simulink model "building_EXAMPLE_v2_r2018b"  (R2018b)
settings: Solver=ode23tb  StartTime=-building.preruntime+8760*3600  StopTime=building.runtime+8760*3600  MaxStep=600  EnableMultiTasking=on
StartFcn:
  | tic
StopFcn:
  | toc
values from neighbouring files (symbols this model uses):
  building = building.add_simulation(1, 'Innsbruck - ERV, 120m3/h, 230 g/h', saveAIB, saveBDB, saveBOUNDARY, saveHVAC, 1)    [work_EXAMPLE_v1.m]
undefined symbols (not defined in the file or in its folder): cp, Dreifach, get_building, p, Qdot_C, Qdot_C_energy, Qdot_H, Qdot_H_energy, Qdot_I_electricity, Qdot_I_electricity_energy, Qdot_I_light, Qdot_I_light_energy, Qdot_I_person, Qdot_I_person_energy, Qdot_S, Qdot_S_energy, Qdot_T_ground, Qdot_T_ground_energy, Qdot_T_neighbour, Qdot_T_neighbour_energy, Qdot_T_opaque, Qdot_T_opaque_energy, Qdot_T_window, Qdot_T_window_energy, Qdot_V_infiltration, Qdot_V_infiltration_energy, Qdot_V_mech, Qdot_V_mech_energy, Qdot_V_window, Qdot_V_window_energy, rho, Tc, Tr, Ts, Wärmeschutzglas, x_CO2, x_H2O, x_VOC
libraries: carnotUIBK x1879, carnot x1
(part 1 of 28)
settings Model: SimulationMode=accelerator  Creator=c8461199  LastModifiedBy=eeb
settings SolverCC: ZeroCrossAlgorithm=Adaptive
settings DataIOCC: SaveOutput=off  SignalLogging=off  DSMLogging=off  VisualizeSimOutput=off  SaveTime=off
settings OptimizationCC: UseDivisionForNetSlopeComputation=on  UseFloatMulNetSlope=on  LifeSpan=inf
settings DebuggingCC: MaxConsecutiveZCsMsg=warning  IgnoredZcDiagnostic=none  AllowSymbolicDim=off  SFUnexpectedBacktrackingDiag=warning  SFNoUnconditionalDefaultTransitionDiag=warning  SFExecutionAtInitializationDiag=none
settings ModelReferenceCC: PropagateSignalLabelsOutOfModel=off
settings SFSimCC: SimUserSources=carlib.c  SimUseLocalCustomCode=off
settings RTWCC: RTWUseLocalCustomCode=off  BuildConfiguration=Faster Runs
settings CodeAppCC: StateflowObjectComments=on
settings GRTTargetCC: TargetLangStandard=C89/C90 (ANSI)
settings ConfigComp: CovMetricSettings=dw  CovHtmlReporting=on  CovSaveCumulativeToWorkspaceVar=on  CovSaveSingleToWorkspaceVar=on  CovExternalEMLEnable=off

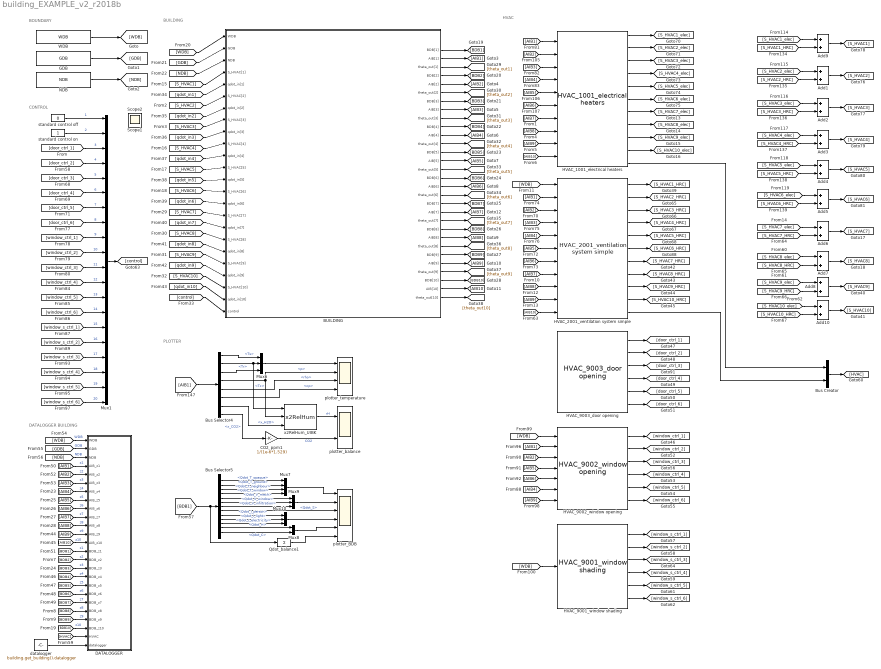
== system building_EXAMPLE_v2_r2018b ==
  note: PLOTTER
  note: DATALOGGER BUILDING
  note: BUILDING
  note: BOUNDARY
  note: HVAC
  note: CONTROL
  Add{1..10} (10 alike) : Sum  Inputs=2
  BUILDING : Subsystem  mask{building=get_building(building)}
      mask prompts: building "BUILDING object"
      mask init:
      | b = building;
      mask Display:
      | plot(-20,-30,120,100,[10,10,90,90,10],[0,50,50,0,0],...
      |     [100,60,40,0],[40,80,80,40],[20,34,34,20,20],[40,40,20,20,40],...
      |     [60,60,40,40],[0,40,40,0],[65,80,80,65,65],[40,40,20,20,40],...
      |     [47,54,54,47,47],[35,35,4,4,35],[45,41],[20,20])
  Bus Creator : BusCreator  Inputs=2
  Bus Selector4 : BusSelector  OutputSignals=Ts,Tc,Tr,p,rho,cp,x_H2O,x_CO2
  Bus Selector5 : BusSelector  OutputSignals=Qdot_T_opaque,Qdot_T_ground,Qdot_T_neighbour,Qdot_T_window,Qdot_V_mech,Qdot_V_window,Qdot_V_infiltration,Qdot_S,Qdot_I_person,Qdot_I_light,Qdot_I_electricity,Qdot_H,Qdot_C
  CO2_ppm1 : Gain  Gain=1/(1e-6*1.529)
  DATALOGGER : Subsystem
  GDB : carnotUIBK/boundary/GDB  building=get_building(building)
  HVAC_1001_electrical heaters : carnotUIBK/HVAC/HVAC_1001_electrical heaters  building=get_building(building)  system=1001
  HVAC_2001_ventilation system simple : carnotUIBK/HVAC/HVAC_2001_ventilation system simple  building=get_building(building)  system=2001
  HVAC_9001_window shading : carnotUIBK/HVAC/HVAC_9001_window shading  building=get_building(building)  system=9001
  HVAC_9002_window opening : carnotUIBK/HVAC/HVAC_9002_window opening  building=get_building(building)  system=9002
  HVAC_9003_door opening : carnotUIBK/HVAC/HVAC_9003_door opening  building=get_building(building)  system=9003
  Mux1 : Mux  Inputs=[1 1 1 1 1 1 1 1 1 1 1 1 1 1 1 1 1 1 1 1]
  Mux10 : Mux  Inputs=3
  Mux6 : Mux  Inputs=3
  Mux7 : Mux
  Mux8 : Mux  Inputs=2
  Mux9 : Mux  Inputs=3
  NDB : carnotUIBK/boundary/NDB  building=get_building(building)
  Qdot_balance1 : Sum  Inputs=1
  WDB : carnotUIBK/boundary/WDB  building=get_building(building)
  datalogger : Constant  Value=building.get_building().datalogger
  plotter_BDB : Scope  NumInputPorts=6
  plotter_balance : Scope  NumInputPorts=2
  plotter_temperature : Scope  NumInputPorts=4
  standard control off : Constant  Value=0
  standard control on : Constant
  x2RelHum_UIBK : carnot/Basic/Material_Properties/x2RelHum
  Scope1 : Scope
  Scope2 : Scope
  wires:
  WDB/1 -> [WDB]
  GDB/1 -> [GDB]
  NDB/1 -> [NDB]
  [WDB] -> BUILDING/1(WDB)
  [GDB] -> BUILDING/2(GDB)
  [NDB] -> BUILDING/3(NDB)
  BUILDING/2(AIB[1]) -> [AIB1]
  BUILDING/5(AIB[2]) -> [AIB2]
  BUILDING/8(AIB[3]) -> [AIB3]
  BUILDING/11(AIB[4]) -> [AIB4]
  BUILDING/14(AIB[5]) -> [AIB5]
  BUILDING/17(AIB[6]) -> [AIB6]
  BUILDING/29(AIB[10]) -> [AIB10]
  BUILDING/26(AIB[9]) -> [AIB9]
  BUILDING/23(AIB[8]) -> [AIB8]
  BUILDING/20(AIB[7]) -> [AIB7]
  [S_HVAC5] -> BUILDING/12(S_HVAC[5])
  [S_HVAC4] -> BUILDING/10(S_HVAC[4])
  [S_HVAC1] -> BUILDING/4(S_HVAC[1])
  [S_HVAC2] -> BUILDING/6(S_HVAC[2])
  [S_HVAC3] -> BUILDING/8(S_HVAC[3])
  [S_HVAC6] -> BUILDING/14(S_HVAC[6])
  [S_HVAC10] -> BUILDING/22(S_HVAC[10])
  [S_HVAC9] -> BUILDING/20(S_HVAC[9])
  [S_HVAC8] -> BUILDING/18(S_HVAC[8])
  [S_HVAC7] -> BUILDING/16(S_HVAC[7])
  [control] -> BUILDING/24(control)
  BUILDING/1(BDB[1]) -> [BDB1]
  BUILDING/28(BDB[10]) -> [BDB10]
  BUILDING/4(BDB[2]) -> [BDB2]
  BUILDING/7(BDB[3]) -> [BDB3]
  BUILDING/10(BDB[4]) -> [BDB4]
  BUILDING/13(BDB[5]) -> [BDB5]
  BUILDING/16(BDB[6]) -> [BDB6]
  BUILDING/19(BDB[7]) -> [BDB7]
  BUILDING/22(BDB[8]) -> [BDB8]
  BUILDING/25(BDB[9]) -> [BDB9]
  [qdot_in1] -> BUILDING/5(qdot_in[1])
  [qdot_in9] -> BUILDING/21(qdot_in[9])
  [qdot_in10] -> BUILDING/23(qdot_in[10])
  [qdot_in8] -> BUILDING/19(qdot_in[8])
  [qdot_in7] -> BUILDING/17(qdot_in[7])
  [qdot_in6] -> BUILDING/15(qdot_in[6])
  [qdot_in4] -> BUILDING/11(qdot_in[4])
  [qdot_in5] -> BUILDING/13(qdot_in[5])
  [qdot_in3] -> BUILDING/9(qdot_in[3])
  [qdot_in2] -> BUILDING/7(qdot_in[2])
  BUILDING/3(theta_out[1]) -> [theta_out1]
  BUILDING/30(theta_out[10]) -> [theta_out10]
  BUILDING/27(theta_out[9]) -> [theta_out9]
  BUILDING/24(theta_out[8]) -> [theta_out8]
  BUILDING/21(theta_out[7]) -> [theta_out7]
  BUILDING/18(theta_out[6]) -> [theta_out6]
  BUILDING/15(theta_out[5]) -> [theta_out5]
  BUILDING/12(theta_out[4]) -> [theta_out4]
  BUILDING/9(theta_out[3]) -> [theta_out3]
  BUILDING/6(theta_out[2]) -> [theta_out2]
  datalogger/1 -> DATALOGGER/25(datalogger)
  [AIB1] -> DATALOGGER/4(AIB_z1)  "z1"
  [WDB] -> DATALOGGER/1(WDB)  "WDB"
  [GDB] -> DATALOGGER/2(GDB)  "GDB"
  [NDB] -> DATALOGGER/3(NDB)  "NDB"
  [AIB2] -> DATALOGGER/5(AIB_z2)  "z2"
  [AIB3] -> DATALOGGER/6(AIB_z3)  "z3"
  [AIB4] -> DATALOGGER/7(AIB_z4)  "z4"
  [AIB5] -> DATALOGGER/8(AIB_z5)  "z5"
  [AIB6] -> DATALOGGER/9(AIB_z6)  "z6"
  [AIB7] -> DATALOGGER/10(AIB_z7)  "z7"
  [AIB8] -> DATALOGGER/11(AIB_z8)  "z8"
  [AIB9] -> DATALOGGER/12(AIB_z9)  "z9"
  [AIB10] -> DATALOGGER/13(AIB_z10)  "z10"
  [BDB1] -> DATALOGGER/14(BDB_z1)  "z1"
  [BDB2] -> DATALOGGER/15(BDB_z2)  "z2"
  [BDB3] -> DATALOGGER/16(BDB_z3)  "z3"
  [BDB4] -> DATALOGGER/17(BDB_z4)  "z4"
  [BDB5] -> DATALOGGER/18(BDB_z5)  "z5"
  [BDB6] -> DATALOGGER/19(BDB_z6)  "z6"
  [BDB7] -> DATALOGGER/20(BDB_z7)  "z7"
  [BDB8] -> DATALOGGER/21(BDB_z8)  "z8"
  [BDB9] -> DATALOGGER/22(BDB_z9)  "z9"
  [BDB10] -> DATALOGGER/23(BDB_z10)  "z10"
  Bus Selector4/4 -> x2RelHum_UIBK/2, plotter_temperature/2  "<p>"
  Bus Selector4/1 -> Mux6/1  "<Ts>"
  Bus Selector4/2 -> x2RelHum_UIBK/1, Mux6/2  "<Tc>"
  Bus Selector4/3 -> Mux6/3  "<Tr>"
  Mux6/1 -> plotter_temperature/1
  Bus Selector4/5 -> plotter_temperature/3  "<rho>"
  Bus Selector4/6 -> plotter_temperature/4  "<cp>"
  Bus Selector4/8 -> CO2_ppm1/1  "<x_CO2>"
  CO2_ppm1/1 -> plotter_balance/2  "CO2"
  Bus Selector4/7 -> x2RelHum_UIBK/3  "<x_H2O>"
  x2RelHum_UIBK/1 -> plotter_balance/1  "rH"
  Bus Selector5/6 -> Mux9/2  "<Qdot_V_window>"
  Bus Selector5/5 -> Mux9/1  "<Qdot_V_mech>"
  Bus Selector5/4 -> Mux7/4  "<Qdot_T_window>"
  Bus Selector5/3 -> Mux7/3  "<Qdot_T_neighbour>"
  Bus Selector5/2 -> Mux7/2  "<Qdot_T_ground>"
  Bus Selector5/1 -> Mux7/1  "<Qdot_T_opaque>"
  Bus Selector5/7 -> Mux9/3  "<Qdot_V_infiltration>"
  Bus Selector5/8 -> plotter_BDB/3  "<Qdot_S>"
  Bus Selector5/9 -> Mux10/1  "<Qdot_I_person>"
  Bus Selector5/10 -> Mux10/2  "<Qdot_I_light>"
  Bus Selector5/11 -> Mux10/3  "<Qdot_I_electricity>"
  Mux7/1 -> plotter_BDB/1
  [BDB1] -> Qdot_balance1/1, Bus Selector5/1
  Mux9/1 -> plotter_BDB/2
  Mux10/1 -> plotter_BDB/4
  Bus Selector5/12 -> Mux8/1  "<Qdot_H>"
  Bus Selector5/13 -> Mux8/2  "<Qdot_C>"
  Mux8/1 -> plotter_BDB/5
  Qdot_balance1/1 -> plotter_BDB/6
  [AIB1] -> Bus Selector4/1
  [HVAC] -> DATALOGGER/24(HVAC)
  Add4/1 -> [S_HVAC5]
  Add3/1 -> [S_HVAC4]
  Add2/1 -> [S_HVAC3]
  Add5/1 -> [S_HVAC6]
  Add9/1 -> [S_HVAC1]
  Add1/1 -> [S_HVAC2]
  [AIB1] -> HVAC_1001_electrical heaters/1
  [AIB2] -> HVAC_1001_electrical heaters/2
  [AIB3] -> HVAC_1001_electrical heaters/3
  [AIB4] -> HVAC_1001_electrical heaters/4
  [AIB5] -> HVAC_1001_electrical heaters/5
  [AIB6] -> HVAC_1001_electrical heaters/6
  HVAC_1001_electrical heaters/1 -> [S_HVAC1_elec]
  HVAC_1001_electrical heaters/6 -> [S_HVAC6_elec]
  HVAC_1001_electrical heaters/3 -> [S_HVAC3_elec]
  HVAC_1001_electrical heaters/4 -> [S_HVAC4_elec]
  HVAC_1001_electrical heaters/2 -> [S_HVAC2_elec]
  HVAC_1001_electrical heaters/5 -> [S_HVAC5_elec]
  HVAC_1001_electrical heaters/9 -> [S_HVAC9_elec]
  HVAC_1001_electrical heaters/10 -> [S_HVAC10_elec]
  HVAC_1001_electrical heaters/8 -> [S_HVAC8_elec]
  HVAC_1001_electrical heaters/7 -> [S_HVAC7_elec]
  [AIB10] -> HVAC_1001_electrical heaters/10
  [AIB9] -> HVAC_1001_electrical heaters/9
  [AIB8] -> HVAC_1001_electrical heaters/8
  [AIB7] -> HVAC_1001_electrical heaters/7
  [AIB7] -> HVAC_2001_ventilation system simple/8
  [WDB] -> HVAC_2001_ventilation system simple/1
  HVAC_2001_ventilation system simple/7 -> [S_HVAC7_HRC]
  [AIB8] -> HVAC_2001_ventilation system simple/9
  [AIB9] -> HVAC_2001_ventilation system simple/10
  [AIB10] -> HVAC_2001_ventilation system simple/11
  HVAC_2001_ventilation system simple/8 -> [S_HVAC8_HRC]
  HVAC_2001_ventilation system simple/9 -> [S_HVAC9_HRC]
  HVAC_2001_ventilation system simple/10 -> [S_HVAC10_HRC]
  Add8/1 -> [S_HVAC9]
  Add6/1 -> [S_HVAC7]
  Add7/1 -> [S_HVAC8]
  Add10/1 -> [S_HVAC10]
  HVAC_9003_door opening/1 -> [door_ctrl_1]
  HVAC_9003_door opening/2 -> [door_ctrl_2]
  HVAC_9003_door opening/4 -> [door_ctrl_4]
  HVAC_9003_door opening/5 -> [door_ctrl_5]
  HVAC_9003_door opening/6 -> [door_ctrl_6]
  [AIB1] -> HVAC_9002_window opening/2
  HVAC_9002_window opening/1 -> [window_ctrl_1]
  [AIB2] -> HVAC_9002_window opening/3
  [AIB6] -> HVAC_9002_window opening/5
  [AIB4] -> HVAC_9002_window opening/6
  [AIB9] -> HVAC_9002_window opening/7
  HVAC_9002_window opening/2 -> [window_ctrl_2]
  HVAC_9002_window opening/4 -> [window_ctrl_4]
  HVAC_9002_window opening/5 -> [window_ctrl_5]
  HVAC_9002_window opening/6 -> [window_ctrl_6]
  [WDB] -> HVAC_9002_window opening/1
  [WDB] -> HVAC_9001_window shading/1
  standard control off/1 -> Mux1/1  "1"
  Mux1/1 -> [control]
  standard control on/1 -> Mux1/2  "2"
  [window_ctrl_1] -> Mux1/9  "9"
  [window_ctrl_6] -> Mux1/14  "14"
  [window_ctrl_5] -> Mux1/13  "13"
  [window_ctrl_4] -> Mux1/12  "12"
  [window_ctrl_3] -> Mux1/11  "11"
  [window_ctrl_2] -> Mux1/10  "10"
  [door_ctrl_1] -> Mux1/3  "3"
  [door_ctrl_2] -> Mux1/4  "4"
  [door_ctrl_3] -> Mux1/5  "5"
  [door_ctrl_4] -> Mux1/6  "6"
  [door_ctrl_5] -> Mux1/7  "7"
  [door_ctrl_6] -> Mux1/8  "8"
  [window_s_ctrl_1] -> Mux1/15  "15"
  [window_s_ctrl_2] -> Mux1/16  "16"
  [window_s_ctrl_3] -> Mux1/17  "17"
  [window_s_ctrl_4] -> Mux1/18  "18"
  [window_s_ctrl_5] -> Mux1/19  "19"
  [window_s_ctrl_6] -> Mux1/20  "20"
  HVAC_9001_window shading/2 -> [window_s_ctrl_2]
  HVAC_9001_window shading/1 -> [window_s_ctrl_1]
  HVAC_2001_ventilation system simple/1 -> [S_HVAC1_HRC]
  HVAC_2001_ventilation system simple/2 -> [S_HVAC2_HRC]
  HVAC_2001_ventilation system simple/3 -> [S_HVAC3_HRC]
  HVAC_2001_ventilation system simple/4 -> [S_HVAC4_HRC]
  HVAC_2001_ventilation system simple/5 -> [S_HVAC5_HRC]
  HVAC_2001_ventilation system simple/6 -> [S_HVAC6_HRC]
  [AIB6] -> HVAC_2001_ventilation system simple/7
  [AIB5] -> HVAC_2001_ventilation system simple/6
  [AIB4] -> HVAC_2001_ventilation system simple/5
  [AIB3] -> HVAC_2001_ventilation system simple/4
  [AIB2] -> HVAC_2001_ventilation system simple/3
  [AIB1] -> HVAC_2001_ventilation system simple/2
  HVAC_9001_window shading/3 -> [window_s_ctrl_3]
  HVAC_9001_window shading/4 -> [window_s_ctrl_4]
  HVAC_9001_window shading/5 -> [window_s_ctrl_5]
  HVAC_9001_window shading/6 -> [window_s_ctrl_6]
  [AIB5] -> HVAC_9002_window opening/4
  HVAC_9002_window opening/3 -> [window_ctrl_3]
  HVAC_9003_door opening/3 -> [door_ctrl_3]
  [S_HVAC1_elec] -> Add9/1
  [S_HVAC1_HRC] -> Add9/2
  [S_HVAC10_elec] -> Add10/1
  [S_HVAC10_HRC] -> Add10/2
  [S_HVAC9_HRC] -> Add8/2
  [S_HVAC9_elec] -> Add8/1
  [S_HVAC8_HRC] -> Add7/2
  [S_HVAC8_elec] -> Add7/1
  [S_HVAC7_HRC] -> Add6/2
  [S_HVAC7_elec] -> Add6/1
  [S_HVAC6_HRC] -> Add5/2
  [S_HVAC6_elec] -> Add5/1
  [S_HVAC5_HRC] -> Add4/2
  [S_HVAC5_elec] -> Add4/1
  [S_HVAC4_HRC] -> Add3/2
  [S_HVAC4_elec] -> Add3/1
  [S_HVAC3_HRC] -> Add2/2
  [S_HVAC3_elec] -> Add2/1
  [S_HVAC2_HRC] -> Add1/2
  [S_HVAC2_elec] -> Add1/1
  Bus Creator/1 -> [HVAC]
  HVAC_1001_electrical heaters/11 -> Bus Creator/1
  HVAC_2001_ventilation system simple/11 -> Bus Creator/2
